simulink model "inverted_pendulum_sim"  (R2021a)
settings: Solver=VariableStepAuto  StartTime=0.0  StopTime=5  RelTol=1e-3
values from neighbouring files (symbols this model uses):
  g = 9.8    [inverted_pendulum.m]
  L = 0.12    [inverted_pendulum.m]
  m = 0.017    [inverted_pendulum.m]
  M = 0.07    [inverted_pendulum.m]
  Mm = 20*0.001    (= 0.02)    [inverted_pendulum.m]
  R = 0.065    [inverted_pendulum.m]
  Rm = 26.3/2*0.01    (= 0.1315)    [inverted_pendulum.m]
  theta1_ini = pi*(90)/180    (= 1.57079632679)    [inverted_pendulum.m]
libraries: pid_lib x1
settings Model: Creator=18214  LastModifiedBy=18214

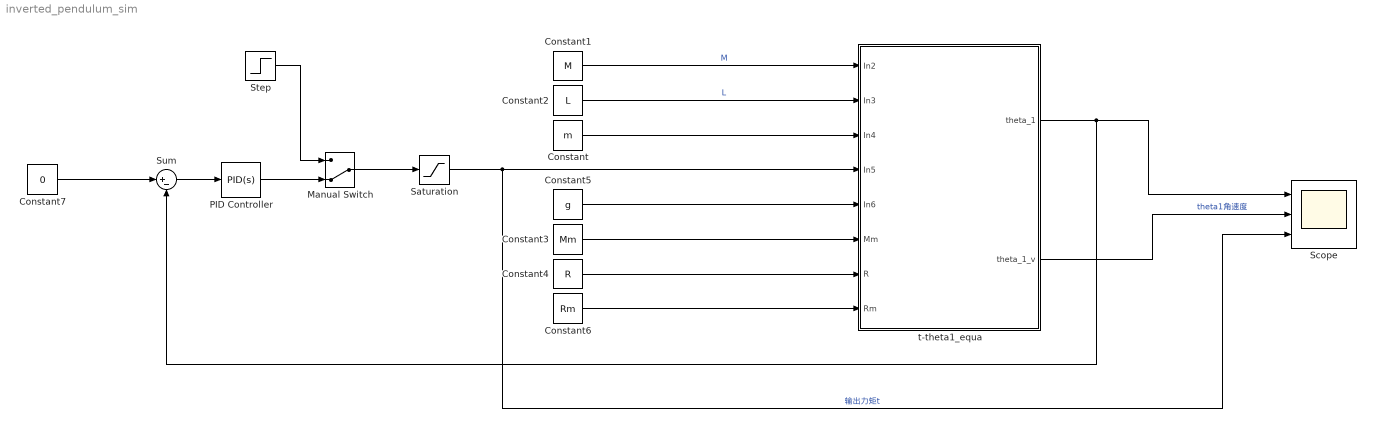
== system inverted_pendulum_sim ==
  Constant : Constant  Value=m
  Constant1 : Constant  Value=M
  Constant2 : Constant  Value=L
  Constant3 : Constant  Value=Mm
  Constant4 : Constant  Value=R
  Constant5 : Constant  Value=g
  Constant6 : Constant  Value=Rm
  Constant7 : Constant  Value=0
  Manual Switch : ManualSwitch  CurrentSetting=0
  PID Controller : pid_lib/PID Controller  Controller=PID  Form=Parallel  TimeDomain=Continuous-time  UseExternalTs=off  SampleTime=-1  IntegratorMethod=Forward Euler  FilterMethod=Forward Euler  ControllerParametersSource=internal  P=0.116  I=0  D=0.005  UseFilter=on  N=100  TunerSelectOption=Transfer Function Based (PID Tuner App)  InitialConditionSource=internal  InitialConditionForIntegrator=0  InitialConditionForFilter=0  DifferentiatorICPrevScaledInput=0  ExternalReset=none  TrackingMode=off  Kt=1  LimitOutput=off  SatLimitsSource=internal  UpperSaturationLimit=inf  LowerSaturationLimit=-inf  LinearizeAsGain=on  AntiWindupMode=none  Kb=1  POutMin=[]  POutMax=[]  IOutMin=[]  IOutMax=[]  DOutMin=[]  DOutMax=[]  NOutMin=[]  NOutMax=[]  SumOutMin=[]  SumOutMax=[]  SaturationOutMin=[]  SaturationOutMax=[]  PParamMin=[]  PParamMax=[]  IParamMin=[]  IParamMax=[]  DParamMin=[]  DParamMax=[]  NParamMin=[]  NParamMax=[]  KbParamMin=[]  KbParamMax=[]  KtParamMin=[]  KtParamMax=[]  KbOutMin=[]  KbOutMax=[]  KtOutMin=[]  KtOutMax=[]  IntegratorOutMin=[]  IntegratorOutMax=[]  FilterOutMin=[]  FilterOutMax=[]  SumI1OutMin=[]  SumI1OutMax=[]  SumI2OutMin=[]  SumI2OutMax=[]  SumI3OutMin=[]  SumI3OutMax=[]  SumI4OutMin=[]  SumI4OutMax=[]  SumDOutMin=[]  SumDOutMax=[]  DifferentiatorOutMin=[]  DifferentiatorOutMax=[]  FilterDiffOutCoefMin=[]  FilterDiffOutCoefMax=[]  ReciprocalOutMin=[]  ReciprocalOutMax=[]  SumDenOutMin=[]  SumDenOutMax=[]  SumNumOutMin=[]  SumNumOutMax=[]  DivideOutMin=[]  DivideOutMax=[]  UdiffTsProdOutMin=[]  UdiffTsProdOutMax=[]  NTsProdOutMin=[]  NTsProdOutMax=[]  UintegralTsProdOutMin=[]  UintegralTsProdOutMax=[]  UngainTsProdOutMin=[]  UngainTsProdOutMax=[]  IntegratorContinuousStateAttributes=''  IntegratorStateMustResolveToSignalObject=off  IntegratorRTWStateStorageClass=Auto  FilterContinuousStateAttributes=''  FilterStateMustResolveToSignalObject=off  FilterRTWStateStorageClass=Auto  ParallelPVariant=InternalParameters  IdealPVariant=Disabled  IVariant=InternalParameters  DVariant=InternalParameters  IntegratorVariant=Continuous  SatVariant=Disabled  AWVariant=Passthrough  PCopyVariant=Disabled  TRVariant=Disabled  FdbkBlocksVariant=Forward  IdealPFdbkVariant=Disabled  SatFdbkVariant=Disabled  DerivativeFilterVariant=ContFilter  NVariant=InternalParameters  NCopyVariant=Disabled  FilterICVariant=InternalICsFilter  IntegratorICVariant=InternalICs  ExternalResetVariant=Disabled  TRSumVariant=Passthrough  SumFdbkVariant=Disabled  SumVariant=Sum_PID  TsampFilterVariant=InternalTs  TsampNgainVariant=Passthrough  TsampIntegralVariant=Passthrough  ExternalSaturationOutDataTypeStr=Inherit: Same as second input
  Saturation : Saturate  UpperLimit=inf  LowerLimit=-inf
  Scope : Scope  NumInputPorts=3
  Step : Step  After=0  SampleTime=0
  Sum : Sum  Inputs=|+-
  t-theta1_equa : Subsystem
  wires:
  Constant1/1 -> t-theta1_equa/1(In2)  "M"
  Constant2/1 -> t-theta1_equa/2(In3)  "L"
  Constant/1 -> t-theta1_equa/3(In4)
  Constant5/1 -> t-theta1_equa/5(In6)
  t-theta1_equa/1(theta_1) -> Scope/1, Sum/2
  t-theta1_equa/2(theta_1_v) -> Scope/2  "theta1角速度"
  Saturation/1 -> Scope/3, t-theta1_equa/4(In5)  "输出力矩t"
  Manual Switch/1 -> Saturation/1
  Constant3/1 -> t-theta1_equa/6(Mm)
  Constant4/1 -> t-theta1_equa/7(R)
  Constant6/1 -> t-theta1_equa/8(Rm)
  Sum/1 -> PID Controller/1
  Constant7/1 -> Sum/1
  PID Controller/1 -> Manual Switch/2
  Step/1 -> Manual Switch/1

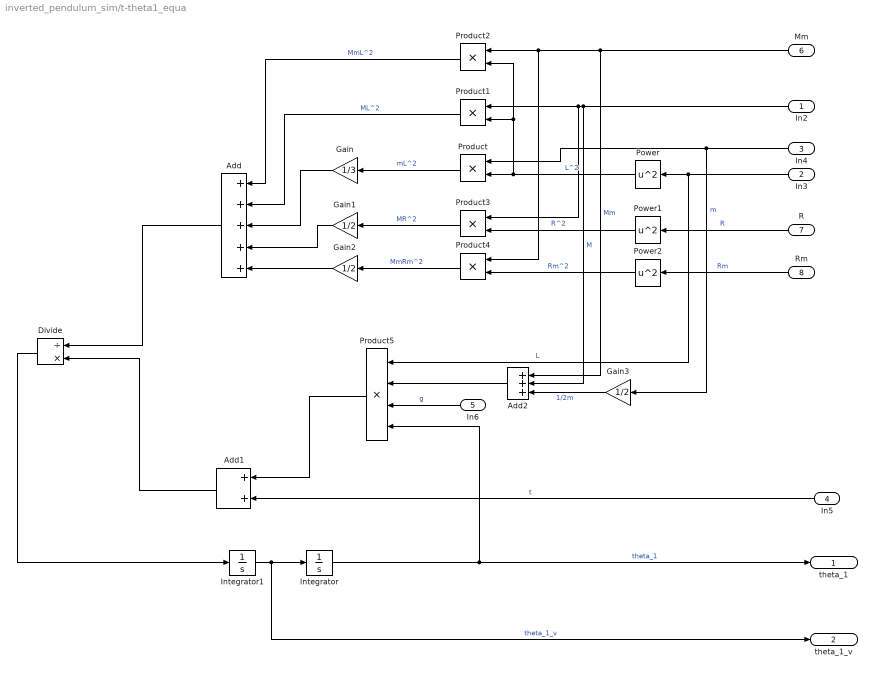
== system inverted_pendulum_sim/t-theta1_equa ==
  In2 : Inport
  In3 : Inport  Port=2
  In4 : Inport  Port=3
  In5 : Inport  Port=4
  In6 : Inport  Port=5
  Mm : Inport  Port=6
  R : Inport  Port=7
  Rm : Inport  Port=8
  Add : Sum  Inputs=+++++
  Add1 : Sum
  Add2 : Sum  Inputs=+++
  Divide : Product  Inputs=/*
  Gain : Gain  Gain=1/3
  Gain1 : Gain  Gain=1/2
  Gain2 : Gain  Gain=1/2
  Gain3 : Gain  Gain=1/2
  Integrator : Integrator  InitialCondition=theta1_ini  LowerSaturationLimit=-pi
  Integrator1 : Integrator
  Power : Math  Operator=square  SaturateOnIntegerOverflow=on
  Power1 : Math  Operator=square  SaturateOnIntegerOverflow=on
  Power2 : Math  Operator=square  SaturateOnIntegerOverflow=on
  Product{,1..4} (5 alike) : Product
  Product5 : Product  Inputs=4
  theta_1 : Outport
  theta_1_v : Outport  Port=2
  wires:
  Integrator/1 -> Product5/4, theta_1/1  "theta_1"
  Integrator1/1 -> theta_1_v/1, Integrator/1  "theta_1_v"
  Mm/1 -> Product4/1, Product2/1, Add2/1  "Mm"
  R/1 -> Power1/1  "R"
  Rm/1 -> Power2/1  "Rm"
  In3/1 -> Product5/1, Power/1  "L"
  Power/1 -> Product2/2, Product1/2, Product/2  "L^2"
  In4/1 -> Product/1, Gain3/1  "m"
  Product/1 -> Gain/1  "mL^2"
  In2/1 -> Product1/1, Product3/1, Add2/2  "M"
  Product1/1 -> Add/2  "ML^2"
  Product2/1 -> Add/1  "MmL^2"
  Power1/1 -> Product3/2  "R^2"
  Power2/1 -> Product4/2  "Rm^2"
  Product3/1 -> Gain1/1  "MR^2"
  Product4/1 -> Gain2/1  "MmRm^2"
  Gain2/1 -> Add/5
  Gain1/1 -> Add/4
  Gain/1 -> Add/3
  Add/1 -> Divide/1
  Add1/1 -> Divide/2
  In5/1 -> Add1/2  "t"
  Gain3/1 -> Add2/3  "1/2m"
  Add2/1 -> Product5/2
  In6/1 -> Product5/3  "g"
  Divide/1 -> Integrator1/1
  Product5/1 -> Add1/1
